simulink model "Thirtybussys"  (R2023b)
settings: Solver=VariableStepAuto  StartTime=0.0  StopTime=1  RelTol=1e-3
libraries: spsFourierLib x60, spsThreePhaseSeriesRLCBranchLib x41, spsThreePhaseVIMeasurementLib x30, spsPower3phInstantaneousLib x30, spsThreePhaseSeriesRLCLoadLib x21, spsThreePhaseSourceLib x6, spsThreePhaseTransformerTwoWindingsLib x6, spsThreePhaseFaultLib x1, sps_lib x1
(part 2 of 2)

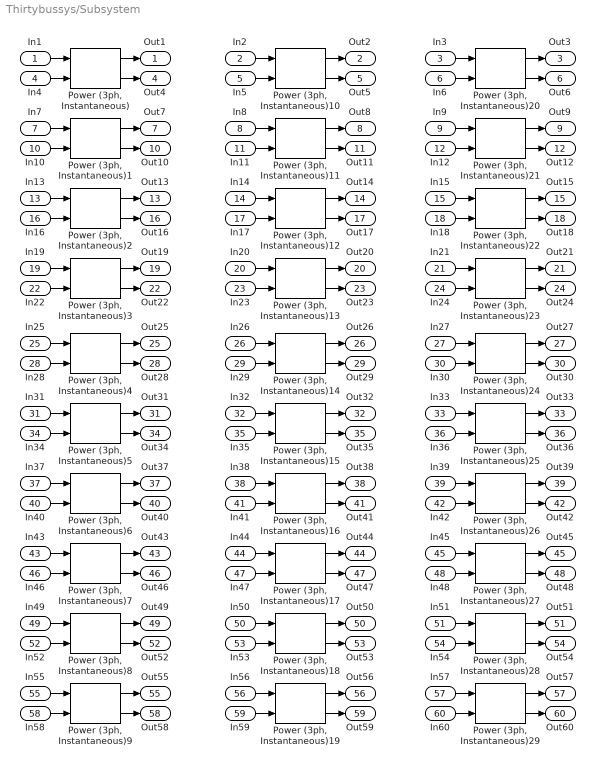
== system Thirtybussys/Subsystem ==
  In1 : Inport
  In2 : Inport  Port=2
  In3 : Inport  Port=3
  In4 : Inport  Port=4
  In5 : Inport  Port=5
  In6 : Inport  Port=6
  In7 : Inport  Port=7
  In8 : Inport  Port=8
  In9 : Inport  Port=9
  In10 : Inport  Port=10
  In11 : Inport  Port=11
  In12 : Inport  Port=12
  In13 : Inport  Port=13
  In14 : Inport  Port=14
  In15 : Inport  Port=15
  In16 : Inport  Port=16
  In17 : Inport  Port=17
  In18 : Inport  Port=18
  In19 : Inport  Port=19
  In20 : Inport  Port=20
  In21 : Inport  Port=21
  In22 : Inport  Port=22
  In23 : Inport  Port=23
  In24 : Inport  Port=24
  In25 : Inport  Port=25
  In26 : Inport  Port=26
  In27 : Inport  Port=27
  In28 : Inport  Port=28
  In29 : Inport  Port=29
  In30 : Inport  Port=30
  In31 : Inport  Port=31
  In32 : Inport  Port=32
  In33 : Inport  Port=33
  In34 : Inport  Port=34
  In35 : Inport  Port=35
  In36 : Inport  Port=36
  In37 : Inport  Port=37
  In38 : Inport  Port=38
  In39 : Inport  Port=39
  In40 : Inport  Port=40
  In41 : Inport  Port=41
  In42 : Inport  Port=42
  In43 : Inport  Port=43
  In44 : Inport  Port=44
  In45 : Inport  Port=45
  In46 : Inport  Port=46
  In47 : Inport  Port=47
  In48 : Inport  Port=48
  In49 : Inport  Port=49
  In50 : Inport  Port=50
  In51 : Inport  Port=51
  In52 : Inport  Port=52
  In53 : Inport  Port=53
  In54 : Inport  Port=54
  In55 : Inport  Port=55
  In56 : Inport  Port=56
  In57 : Inport  Port=57
  In58 : Inport  Port=58
  In59 : Inport  Port=59
  In60 : Inport  Port=60
  Power (3ph, Instantaneous){,1..29} (30 alike) : spsPower3phInstantaneousLib/Power (3ph, Instantaneous)
  Out1 : Outport  VectorParamsAs1DForOutWhenUnconnected=off
  Out2 : Outport  Port=2  VectorParamsAs1DForOutWhenUnconnected=off
  Out3 : Outport  Port=3  VectorParamsAs1DForOutWhenUnconnected=off
  Out4 : Outport  Port=4  VectorParamsAs1DForOutWhenUnconnected=off
  Out5 : Outport  Port=5  VectorParamsAs1DForOutWhenUnconnected=off
  Out6 : Outport  Port=6  VectorParamsAs1DForOutWhenUnconnected=off
  Out7 : Outport  Port=7  VectorParamsAs1DForOutWhenUnconnected=off
  Out8 : Outport  Port=8  VectorParamsAs1DForOutWhenUnconnected=off
  Out9 : Outport  Port=9  VectorParamsAs1DForOutWhenUnconnected=off
  Out10 : Outport  Port=10  VectorParamsAs1DForOutWhenUnconnected=off
  Out11 : Outport  Port=11  VectorParamsAs1DForOutWhenUnconnected=off
  Out12 : Outport  Port=12  VectorParamsAs1DForOutWhenUnconnected=off
  Out13 : Outport  Port=13  VectorParamsAs1DForOutWhenUnconnected=off
  Out14 : Outport  Port=14  VectorParamsAs1DForOutWhenUnconnected=off
  Out15 : Outport  Port=15  VectorParamsAs1DForOutWhenUnconnected=off
  Out16 : Outport  Port=16  VectorParamsAs1DForOutWhenUnconnected=off
  Out17 : Outport  Port=17  VectorParamsAs1DForOutWhenUnconnected=off
  Out18 : Outport  Port=18  VectorParamsAs1DForOutWhenUnconnected=off
  Out19 : Outport  Port=19  VectorParamsAs1DForOutWhenUnconnected=off
  Out20 : Outport  Port=20  VectorParamsAs1DForOutWhenUnconnected=off
  Out21 : Outport  Port=21  VectorParamsAs1DForOutWhenUnconnected=off
  Out22 : Outport  Port=22  VectorParamsAs1DForOutWhenUnconnected=off
  Out23 : Outport  Port=23  VectorParamsAs1DForOutWhenUnconnected=off
  Out24 : Outport  Port=24  VectorParamsAs1DForOutWhenUnconnected=off
  Out25 : Outport  Port=25  VectorParamsAs1DForOutWhenUnconnected=off
  Out26 : Outport  Port=26  VectorParamsAs1DForOutWhenUnconnected=off
  Out27 : Outport  Port=27  VectorParamsAs1DForOutWhenUnconnected=off
  Out28 : Outport  Port=28  VectorParamsAs1DForOutWhenUnconnected=off
  Out29 : Outport  Port=29  VectorParamsAs1DForOutWhenUnconnected=off
  Out30 : Outport  Port=30  VectorParamsAs1DForOutWhenUnconnected=off
  Out31 : Outport  Port=31  VectorParamsAs1DForOutWhenUnconnected=off
  Out32 : Outport  Port=32  VectorParamsAs1DForOutWhenUnconnected=off
  Out33 : Outport  Port=33  VectorParamsAs1DForOutWhenUnconnected=off
  Out34 : Outport  Port=34  VectorParamsAs1DForOutWhenUnconnected=off
  Out35 : Outport  Port=35  VectorParamsAs1DForOutWhenUnconnected=off
  Out36 : Outport  Port=36  VectorParamsAs1DForOutWhenUnconnected=off
  Out37 : Outport  Port=37  VectorParamsAs1DForOutWhenUnconnected=off
  Out38 : Outport  Port=38  VectorParamsAs1DForOutWhenUnconnected=off
  Out39 : Outport  Port=39  VectorParamsAs1DForOutWhenUnconnected=off
  Out40 : Outport  Port=40  VectorParamsAs1DForOutWhenUnconnected=off
  Out41 : Outport  Port=41  VectorParamsAs1DForOutWhenUnconnected=off
  Out42 : Outport  Port=42  VectorParamsAs1DForOutWhenUnconnected=off
  Out43 : Outport  Port=43  VectorParamsAs1DForOutWhenUnconnected=off
  Out44 : Outport  Port=44  VectorParamsAs1DForOutWhenUnconnected=off
  Out45 : Outport  Port=45  VectorParamsAs1DForOutWhenUnconnected=off
  Out46 : Outport  Port=46  VectorParamsAs1DForOutWhenUnconnected=off
  Out47 : Outport  Port=47  VectorParamsAs1DForOutWhenUnconnected=off
  Out48 : Outport  Port=48  VectorParamsAs1DForOutWhenUnconnected=off
  Out49 : Outport  Port=49  VectorParamsAs1DForOutWhenUnconnected=off
  Out50 : Outport  Port=50  VectorParamsAs1DForOutWhenUnconnected=off
  Out51 : Outport  Port=51  VectorParamsAs1DForOutWhenUnconnected=off
  Out52 : Outport  Port=52  VectorParamsAs1DForOutWhenUnconnected=off
  Out53 : Outport  Port=53  VectorParamsAs1DForOutWhenUnconnected=off
  Out54 : Outport  Port=54  VectorParamsAs1DForOutWhenUnconnected=off
  Out55 : Outport  Port=55  VectorParamsAs1DForOutWhenUnconnected=off
  Out56 : Outport  Port=56  VectorParamsAs1DForOutWhenUnconnected=off
  Out57 : Outport  Port=57  VectorParamsAs1DForOutWhenUnconnected=off
  Out58 : Outport  Port=58  VectorParamsAs1DForOutWhenUnconnected=off
  Out59 : Outport  Port=59  VectorParamsAs1DForOutWhenUnconnected=off
  Out60 : Outport  Port=60  VectorParamsAs1DForOutWhenUnconnected=off
  wires:
  In20/1 -> "Power (3ph, Instantaneous)13"/1
  "Power (3ph, Instantaneous)4"/1 -> Out25/1
  In18/1 -> "Power (3ph, Instantaneous)22"/2
  "Power (3ph, Instantaneous)10"/1 -> Out2/1
  "Power (3ph, Instantaneous)11"/2 -> Out11/1
  In48/1 -> "Power (3ph, Instantaneous)27"/2
  "Power (3ph, Instantaneous)28"/2 -> Out54/1
  In25/1 -> "Power (3ph, Instantaneous)4"/1
  In41/1 -> "Power (3ph, Instantaneous)16"/2
  "Power (3ph, Instantaneous)28"/1 -> Out51/1
  In11/1 -> "Power (3ph, Instantaneous)11"/2
  In36/1 -> "Power (3ph, Instantaneous)25"/2
  "Power (3ph, Instantaneous)21"/1 -> Out9/1
  In46/1 -> "Power (3ph, Instantaneous)7"/2
  In38/1 -> "Power (3ph, Instantaneous)16"/1
  "Power (3ph, Instantaneous)14"/2 -> Out29/1
  "Power (3ph, Instantaneous)20"/2 -> Out6/1
  In23/1 -> "Power (3ph, Instantaneous)13"/2
  "Power (3ph, Instantaneous)13"/2 -> Out23/1
  In17/1 -> "Power (3ph, Instantaneous)12"/2
  "Power (3ph, Instantaneous)17"/2 -> Out47/1
  In47/1 -> "Power (3ph, Instantaneous)17"/2
  In26/1 -> "Power (3ph, Instantaneous)14"/1
  "Power (3ph, Instantaneous)15"/1 -> Out32/1
  In12/1 -> "Power (3ph, Instantaneous)21"/2
  "Power (3ph, Instantaneous)8"/2 -> Out52/1
  "Power (3ph, Instantaneous)16"/2 -> Out41/1
  In57/1 -> "Power (3ph, Instantaneous)29"/1
  In35/1 -> "Power (3ph, Instantaneous)15"/2
  In52/1 -> "Power (3ph, Instantaneous)8"/2
  "Power (3ph, Instantaneous)2"/1 -> Out13/1
  In16/1 -> "Power (3ph, Instantaneous)2"/2
  In6/1 -> "Power (3ph, Instantaneous)20"/2
  In29/1 -> "Power (3ph, Instantaneous)14"/2
  In42/1 -> "Power (3ph, Instantaneous)26"/2
  "Power (3ph, Instantaneous)1"/1 -> Out7/1
  In58/1 -> "Power (3ph, Instantaneous)9"/2
  "Power (3ph, Instantaneous)15"/2 -> Out35/1
  In19/1 -> "Power (3ph, Instantaneous)3"/1
  "Power (3ph, Instantaneous)9"/2 -> Out58/1
  In30/1 -> "Power (3ph, Instantaneous)24"/2
  "Power (3ph, Instantaneous)12"/2 -> Out17/1
  "Power (3ph, Instantaneous)24"/2 -> Out30/1
  "Power (3ph, Instantaneous)23"/2 -> Out24/1
  In60/1 -> "Power (3ph, Instantaneous)29"/2
  "Power (3ph, Instantaneous)20"/1 -> Out3/1
  "Power (3ph, Instantaneous)22"/1 -> Out15/1
  In24/1 -> "Power (3ph, Instantaneous)23"/2
  "Power (3ph, Instantaneous)25"/2 -> Out36/1
  In27/1 -> "Power (3ph, Instantaneous)24"/1
  In54/1 -> "Power (3ph, Instantaneous)28"/2
  "Power (3ph, Instantaneous)12"/1 -> Out14/1
  In55/1 -> "Power (3ph, Instantaneous)9"/1
  In22/1 -> "Power (3ph, Instantaneous)3"/2
  "Power (3ph, Instantaneous)2"/2 -> Out16/1
  "Power (3ph, Instantaneous)14"/1 -> Out26/1
  "Power (3ph, Instantaneous)3"/2 -> Out22/1
  "Power (3ph, Instantaneous)26"/2 -> Out42/1
  "Power (3ph, Instantaneous)27"/2 -> Out48/1
  In28/1 -> "Power (3ph, Instantaneous)4"/2
  "Power (3ph, Instantaneous)29"/2 -> Out60/1
  "Power (3ph, Instantaneous)26"/1 -> Out39/1
  "Power (3ph, Instantaneous)23"/1 -> Out21/1
  In7/1 -> "Power (3ph, Instantaneous)1"/1
  "Power (3ph, Instantaneous)7"/2 -> Out46/1
  "Power (3ph, Instantaneous)21"/2 -> Out12/1
  "Power (3ph, Instantaneous)22"/2 -> Out18/1
  In9/1 -> "Power (3ph, Instantaneous)21"/1
  In32/1 -> "Power (3ph, Instantaneous)15"/1
  "Power (3ph, Instantaneous)16"/1 -> Out38/1
  In39/1 -> "Power (3ph, Instantaneous)26"/1
  In15/1 -> "Power (3ph, Instantaneous)22"/1
  In44/1 -> "Power (3ph, Instantaneous)17"/1
  "Power (3ph, Instantaneous)29"/1 -> Out57/1
  "Power (3ph, Instantaneous)24"/1 -> Out27/1
  In21/1 -> "Power (3ph, Instantaneous)23"/1
  In31/1 -> "Power (3ph, Instantaneous)5"/1
  "Power (3ph, Instantaneous)5"/1 -> Out31/1
  In43/1 -> "Power (3ph, Instantaneous)7"/1
  "Power (3ph, Instantaneous)3"/1 -> Out19/1
  "Power (3ph, Instantaneous)6"/1 -> Out37/1
  In37/1 -> "Power (3ph, Instantaneous)6"/1
  In33/1 -> "Power (3ph, Instantaneous)25"/1
  In1/1 -> "Power (3ph, Instantaneous)"/1
  "Power (3ph, Instantaneous)"/1 -> Out1/1
  In50/1 -> "Power (3ph, Instantaneous)18"/1
  "Power (3ph, Instantaneous)25"/1 -> Out33/1
  "Power (3ph, Instantaneous)17"/1 -> Out44/1
  In56/1 -> "Power (3ph, Instantaneous)19"/1
  "Power (3ph, Instantaneous)18"/1 -> Out50/1
  "Power (3ph, Instantaneous)9"/1 -> Out55/1
  "Power (3ph, Instantaneous)7"/1 -> Out43/1
  "Power (3ph, Instantaneous)19"/1 -> Out56/1
  In45/1 -> "Power (3ph, Instantaneous)27"/1
  In2/1 -> "Power (3ph, Instantaneous)10"/1
  In10/1 -> "Power (3ph, Instantaneous)1"/2
  In49/1 -> "Power (3ph, Instantaneous)8"/1
  "Power (3ph, Instantaneous)27"/1 -> Out45/1
  "Power (3ph, Instantaneous)8"/1 -> Out49/1
  "Power (3ph, Instantaneous)13"/1 -> Out20/1
  In14/1 -> "Power (3ph, Instantaneous)12"/1
  In13/1 -> "Power (3ph, Instantaneous)2"/1
  In51/1 -> "Power (3ph, Instantaneous)28"/1
  In3/1 -> "Power (3ph, Instantaneous)20"/1
  In8/1 -> "Power (3ph, Instantaneous)11"/1
  "Power (3ph, Instantaneous)11"/1 -> Out8/1
  "Power (3ph, Instantaneous)"/2 -> Out4/1
  "Power (3ph, Instantaneous)10"/2 -> Out5/1
  "Power (3ph, Instantaneous)4"/2 -> Out28/1
  "Power (3ph, Instantaneous)6"/2 -> Out40/1
  "Power (3ph, Instantaneous)5"/2 -> Out34/1
  "Power (3ph, Instantaneous)18"/2 -> Out53/1
  "Power (3ph, Instantaneous)19"/2 -> Out59/1
  In40/1 -> "Power (3ph, Instantaneous)6"/2
  In53/1 -> "Power (3ph, Instantaneous)18"/2
  In34/1 -> "Power (3ph, Instantaneous)5"/2
  In4/1 -> "Power (3ph, Instantaneous)"/2
  In59/1 -> "Power (3ph, Instantaneous)19"/2
  "Power (3ph, Instantaneous)1"/2 -> Out10/1
  In5/1 -> "Power (3ph, Instantaneous)10"/2

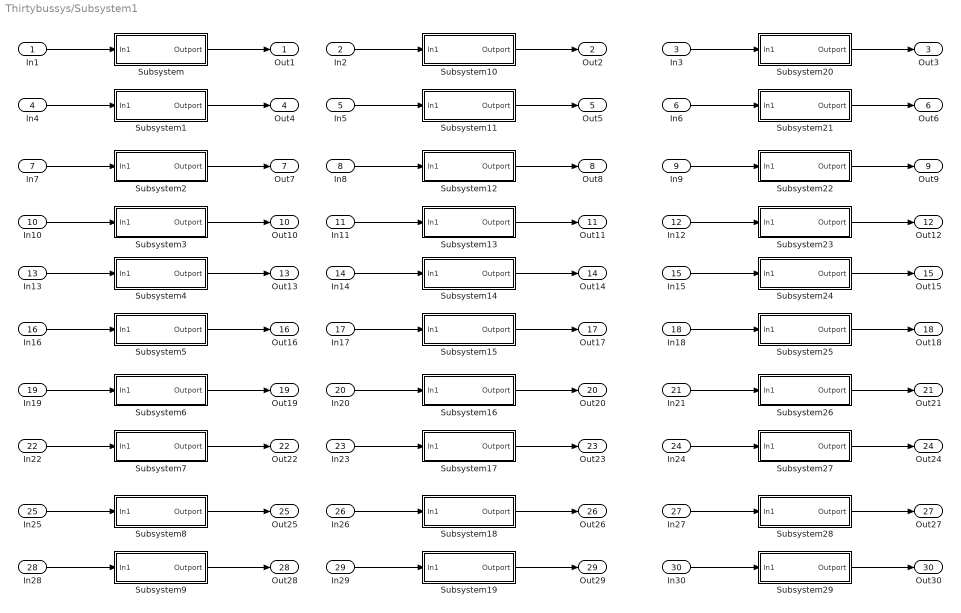
== system Thirtybussys/Subsystem1 ==
  In1 : Inport
  In2 : Inport  Port=2
  In3 : Inport  Port=3
  In4 : Inport  Port=4
  In5 : Inport  Port=5
  In6 : Inport  Port=6
  In7 : Inport  Port=7
  In8 : Inport  Port=8
  In9 : Inport  Port=9
  In10 : Inport  Port=10
  In11 : Inport  Port=11
  In12 : Inport  Port=12
  In13 : Inport  Port=13
  In14 : Inport  Port=14
  In15 : Inport  Port=15
  In16 : Inport  Port=16
  In17 : Inport  Port=17
  In18 : Inport  Port=18
  In19 : Inport  Port=19
  In20 : Inport  Port=20
  In21 : Inport  Port=21
  In22 : Inport  Port=22
  In23 : Inport  Port=23
  In24 : Inport  Port=24
  In25 : Inport  Port=25
  In26 : Inport  Port=26
  In27 : Inport  Port=27
  In28 : Inport  Port=28
  In29 : Inport  Port=29
  In30 : Inport  Port=30
  Subsystem : Subsystem
  Subsystem1 : Subsystem
  Subsystem10 : Subsystem
  Subsystem11 : Subsystem
  Subsystem12 : Subsystem
  Subsystem13 : Subsystem
  Subsystem14 : Subsystem
  Subsystem15 : Subsystem
  Subsystem16 : Subsystem
  Subsystem17 : Subsystem
  Subsystem18 : Subsystem
  Subsystem19 : Subsystem
  Subsystem2 : Subsystem
  Subsystem20 : Subsystem
  Subsystem21 : Subsystem
  Subsystem22 : Subsystem
  Subsystem23 : Subsystem
  Subsystem24 : Subsystem
  Subsystem25 : Subsystem
  Subsystem26 : Subsystem
  Subsystem27 : Subsystem
  Subsystem28 : Subsystem
  Subsystem29 : Subsystem
  Subsystem3 : Subsystem
  Subsystem4 : Subsystem
  Subsystem5 : Subsystem
  Subsystem6 : Subsystem
  Subsystem7 : Subsystem
  Subsystem8 : Subsystem
  Subsystem9 : Subsystem
  Out1 : Outport  VectorParamsAs1DForOutWhenUnconnected=off
  Out2 : Outport  Port=2  VectorParamsAs1DForOutWhenUnconnected=off
  Out3 : Outport  Port=3  VectorParamsAs1DForOutWhenUnconnected=off
  Out4 : Outport  Port=4  VectorParamsAs1DForOutWhenUnconnected=off
  Out5 : Outport  Port=5  VectorParamsAs1DForOutWhenUnconnected=off
  Out6 : Outport  Port=6  VectorParamsAs1DForOutWhenUnconnected=off
  Out7 : Outport  Port=7  VectorParamsAs1DForOutWhenUnconnected=off
  Out8 : Outport  Port=8  VectorParamsAs1DForOutWhenUnconnected=off
  Out9 : Outport  Port=9  VectorParamsAs1DForOutWhenUnconnected=off
  Out10 : Outport  Port=10  VectorParamsAs1DForOutWhenUnconnected=off
  Out11 : Outport  Port=11  VectorParamsAs1DForOutWhenUnconnected=off
  Out12 : Outport  Port=12  VectorParamsAs1DForOutWhenUnconnected=off
  Out13 : Outport  Port=13  VectorParamsAs1DForOutWhenUnconnected=off
  Out14 : Outport  Port=14  VectorParamsAs1DForOutWhenUnconnected=off
  Out15 : Outport  Port=15  VectorParamsAs1DForOutWhenUnconnected=off
  Out16 : Outport  Port=16  VectorParamsAs1DForOutWhenUnconnected=off
  Out17 : Outport  Port=17  VectorParamsAs1DForOutWhenUnconnected=off
  Out18 : Outport  Port=18  VectorParamsAs1DForOutWhenUnconnected=off
  Out19 : Outport  Port=19  VectorParamsAs1DForOutWhenUnconnected=off
  Out20 : Outport  Port=20  VectorParamsAs1DForOutWhenUnconnected=off
  Out21 : Outport  Port=21  VectorParamsAs1DForOutWhenUnconnected=off
  Out22 : Outport  Port=22  VectorParamsAs1DForOutWhenUnconnected=off
  Out23 : Outport  Port=23  VectorParamsAs1DForOutWhenUnconnected=off
  Out24 : Outport  Port=24  VectorParamsAs1DForOutWhenUnconnected=off
  Out25 : Outport  Port=25  VectorParamsAs1DForOutWhenUnconnected=off
  Out26 : Outport  Port=26  VectorParamsAs1DForOutWhenUnconnected=off
  Out27 : Outport  Port=27  VectorParamsAs1DForOutWhenUnconnected=off
  Out28 : Outport  Port=28  VectorParamsAs1DForOutWhenUnconnected=off
  Out29 : Outport  Port=29  VectorParamsAs1DForOutWhenUnconnected=off
  Out30 : Outport  Port=30  VectorParamsAs1DForOutWhenUnconnected=off
  wires:
  Subsystem/1(Outport) -> Out1/1
  Subsystem6/1(Outport) -> Out19/1
  In28/1 -> Subsystem9/1(In1)
  In14/1 -> Subsystem14/1(In1)
  In29/1 -> Subsystem19/1(In1)
  Subsystem7/1(Outport) -> Out22/1
  In11/1 -> Subsystem13/1(In1)
  Subsystem17/1(Outport) -> Out23/1
  In5/1 -> Subsystem11/1(In1)
  Subsystem16/1(Outport) -> Out20/1
  In19/1 -> Subsystem6/1(In1)
  In8/1 -> Subsystem12/1(In1)
  In23/1 -> Subsystem17/1(In1)
  Subsystem18/1(Outport) -> Out26/1
  In25/1 -> Subsystem8/1(In1)
  In10/1 -> Subsystem3/1(In1)
  Subsystem28/1(Outport) -> Out27/1
  In7/1 -> Subsystem2/1(In1)
  Subsystem29/1(Outport) -> Out30/1
  Subsystem15/1(Outport) -> Out17/1
  In26/1 -> Subsystem18/1(In1)
  Subsystem25/1(Outport) -> Out18/1
  In15/1 -> Subsystem24/1(In1)
  Subsystem24/1(Outport) -> Out15/1
  In21/1 -> Subsystem26/1(In1)
  In24/1 -> Subsystem27/1(In1)
  Subsystem1/1(Outport) -> Out4/1
  Subsystem23/1(Outport) -> Out12/1
  Subsystem19/1(Outport) -> Out29/1
  Subsystem13/1(Outport) -> Out11/1
  In3/1 -> Subsystem20/1(In1)
  In12/1 -> Subsystem23/1(In1)
  Subsystem10/1(Outport) -> Out2/1
  In17/1 -> Subsystem15/1(In1)
  In2/1 -> Subsystem10/1(In1)
  Subsystem4/1(Outport) -> Out13/1
  In16/1 -> Subsystem5/1(In1)
  Subsystem14/1(Outport) -> Out14/1
  In13/1 -> Subsystem4/1(In1)
  In18/1 -> Subsystem25/1(In1)
  Subsystem9/1(Outport) -> Out28/1
  Subsystem8/1(Outport) -> Out25/1
  In20/1 -> Subsystem16/1(In1)
  Subsystem20/1(Outport) -> Out3/1
  Subsystem11/1(Outport) -> Out5/1
  Subsystem27/1(Outport) -> Out24/1
  In30/1 -> Subsystem29/1(In1)
  Subsystem2/1(Outport) -> Out7/1
  In22/1 -> Subsystem7/1(In1)
  Subsystem12/1(Outport) -> Out8/1
  Subsystem3/1(Outport) -> Out10/1
  Subsystem21/1(Outport) -> Out6/1
  In9/1 -> Subsystem22/1(In1)
  In4/1 -> Subsystem1/1(In1)
  Subsystem26/1(Outport) -> Out21/1
  Subsystem5/1(Outport) -> Out16/1
  In27/1 -> Subsystem28/1(In1)
  In1/1 -> Subsystem/1(In1)
  In6/1 -> Subsystem21/1(In1)
  Subsystem22/1(Outport) -> Out9/1

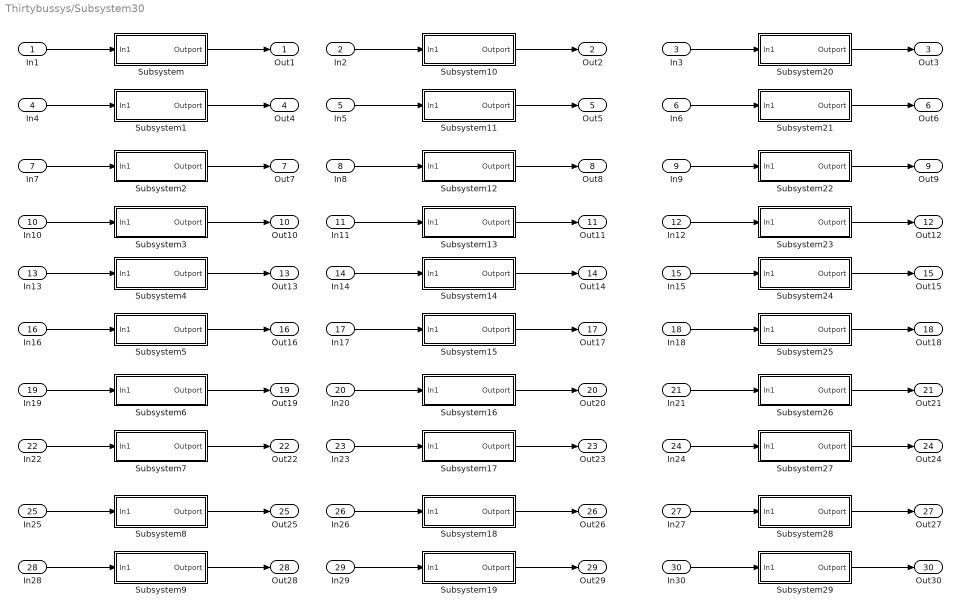
== system Thirtybussys/Subsystem30 ==
  In1 : Inport
  In2 : Inport  Port=2
  In3 : Inport  Port=3
  In4 : Inport  Port=4
  In5 : Inport  Port=5
  In6 : Inport  Port=6
  In7 : Inport  Port=7
  In8 : Inport  Port=8
  In9 : Inport  Port=9
  In10 : Inport  Port=10
  In11 : Inport  Port=11
  In12 : Inport  Port=12
  In13 : Inport  Port=13
  In14 : Inport  Port=14
  In15 : Inport  Port=15
  In16 : Inport  Port=16
  In17 : Inport  Port=17
  In18 : Inport  Port=18
  In19 : Inport  Port=19
  In20 : Inport  Port=20
  In21 : Inport  Port=21
  In22 : Inport  Port=22
  In23 : Inport  Port=23
  In24 : Inport  Port=24
  In25 : Inport  Port=25
  In26 : Inport  Port=26
  In27 : Inport  Port=27
  In28 : Inport  Port=28
  In29 : Inport  Port=29
  In30 : Inport  Port=30
  Subsystem : Subsystem
  Subsystem1 : Subsystem
  Subsystem10 : Subsystem
  Subsystem11 : Subsystem
  Subsystem12 : Subsystem
  Subsystem13 : Subsystem
  Subsystem14 : Subsystem
  Subsystem15 : Subsystem
  Subsystem16 : Subsystem
  Subsystem17 : Subsystem
  Subsystem18 : Subsystem
  Subsystem19 : Subsystem
  Subsystem2 : Subsystem
  Subsystem20 : Subsystem
  Subsystem21 : Subsystem
  Subsystem22 : Subsystem
  Subsystem23 : Subsystem
  Subsystem24 : Subsystem
  Subsystem25 : Subsystem
  Subsystem26 : Subsystem
  Subsystem27 : Subsystem
  Subsystem28 : Subsystem
  Subsystem29 : Subsystem
  Subsystem3 : Subsystem
  Subsystem4 : Subsystem
  Subsystem5 : Subsystem
  Subsystem6 : Subsystem
  Subsystem7 : Subsystem
  Subsystem8 : Subsystem
  Subsystem9 : Subsystem
  Out1 : Outport  VectorParamsAs1DForOutWhenUnconnected=off
  Out2 : Outport  Port=2  VectorParamsAs1DForOutWhenUnconnected=off
  Out3 : Outport  Port=3  VectorParamsAs1DForOutWhenUnconnected=off
  Out4 : Outport  Port=4  VectorParamsAs1DForOutWhenUnconnected=off
  Out5 : Outport  Port=5  VectorParamsAs1DForOutWhenUnconnected=off
  Out6 : Outport  Port=6  VectorParamsAs1DForOutWhenUnconnected=off
  Out7 : Outport  Port=7  VectorParamsAs1DForOutWhenUnconnected=off
  Out8 : Outport  Port=8  VectorParamsAs1DForOutWhenUnconnected=off
  Out9 : Outport  Port=9  VectorParamsAs1DForOutWhenUnconnected=off
  Out10 : Outport  Port=10  VectorParamsAs1DForOutWhenUnconnected=off
  Out11 : Outport  Port=11  VectorParamsAs1DForOutWhenUnconnected=off
  Out12 : Outport  Port=12  VectorParamsAs1DForOutWhenUnconnected=off
  Out13 : Outport  Port=13  VectorParamsAs1DForOutWhenUnconnected=off
  Out14 : Outport  Port=14  VectorParamsAs1DForOutWhenUnconnected=off
  Out15 : Outport  Port=15  VectorParamsAs1DForOutWhenUnconnected=off
  Out16 : Outport  Port=16  VectorParamsAs1DForOutWhenUnconnected=off
  Out17 : Outport  Port=17  VectorParamsAs1DForOutWhenUnconnected=off
  Out18 : Outport  Port=18  VectorParamsAs1DForOutWhenUnconnected=off
  Out19 : Outport  Port=19  VectorParamsAs1DForOutWhenUnconnected=off
  Out20 : Outport  Port=20  VectorParamsAs1DForOutWhenUnconnected=off
  Out21 : Outport  Port=21  VectorParamsAs1DForOutWhenUnconnected=off
  Out22 : Outport  Port=22  VectorParamsAs1DForOutWhenUnconnected=off
  Out23 : Outport  Port=23  VectorParamsAs1DForOutWhenUnconnected=off
  Out24 : Outport  Port=24  VectorParamsAs1DForOutWhenUnconnected=off
  Out25 : Outport  Port=25  VectorParamsAs1DForOutWhenUnconnected=off
  Out26 : Outport  Port=26  VectorParamsAs1DForOutWhenUnconnected=off
  Out27 : Outport  Port=27  VectorParamsAs1DForOutWhenUnconnected=off
  Out28 : Outport  Port=28  VectorParamsAs1DForOutWhenUnconnected=off
  Out29 : Outport  Port=29  VectorParamsAs1DForOutWhenUnconnected=off
  Out30 : Outport  Port=30  VectorParamsAs1DForOutWhenUnconnected=off
  wires:
  Subsystem22/1(Outport) -> Out9/1
  In6/1 -> Subsystem21/1(In1)
  In1/1 -> Subsystem/1(In1)
  In27/1 -> Subsystem28/1(In1)
  Subsystem5/1(Outport) -> Out16/1
  Subsystem26/1(Outport) -> Out21/1
  In4/1 -> Subsystem1/1(In1)
  In9/1 -> Subsystem22/1(In1)
  Subsystem21/1(Outport) -> Out6/1
  Subsystem3/1(Outport) -> Out10/1
  Subsystem12/1(Outport) -> Out8/1
  In22/1 -> Subsystem7/1(In1)
  Subsystem2/1(Outport) -> Out7/1
  In30/1 -> Subsystem29/1(In1)
  Subsystem27/1(Outport) -> Out24/1
  Subsystem11/1(Outport) -> Out5/1
  Subsystem20/1(Outport) -> Out3/1
  In20/1 -> Subsystem16/1(In1)
  Subsystem8/1(Outport) -> Out25/1
  Subsystem9/1(Outport) -> Out28/1
  In18/1 -> Subsystem25/1(In1)
  In13/1 -> Subsystem4/1(In1)
  Subsystem14/1(Outport) -> Out14/1
  In16/1 -> Subsystem5/1(In1)
  Subsystem4/1(Outport) -> Out13/1
  In2/1 -> Subsystem10/1(In1)
  In17/1 -> Subsystem15/1(In1)
  Subsystem10/1(Outport) -> Out2/1
  In12/1 -> Subsystem23/1(In1)
  In3/1 -> Subsystem20/1(In1)
  Subsystem13/1(Outport) -> Out11/1
  Subsystem19/1(Outport) -> Out29/1
  Subsystem23/1(Outport) -> Out12/1
  Subsystem1/1(Outport) -> Out4/1
  In24/1 -> Subsystem27/1(In1)
  In21/1 -> Subsystem26/1(In1)
  Subsystem24/1(Outport) -> Out15/1
  In15/1 -> Subsystem24/1(In1)
  Subsystem25/1(Outport) -> Out18/1
  In26/1 -> Subsystem18/1(In1)
  Subsystem15/1(Outport) -> Out17/1
  Subsystem29/1(Outport) -> Out30/1
  In7/1 -> Subsystem2/1(In1)
  Subsystem28/1(Outport) -> Out27/1
  In10/1 -> Subsystem3/1(In1)
  In25/1 -> Subsystem8/1(In1)
  Subsystem18/1(Outport) -> Out26/1
  In23/1 -> Subsystem17/1(In1)
  In8/1 -> Subsystem12/1(In1)
  In19/1 -> Subsystem6/1(In1)
  Subsystem16/1(Outport) -> Out20/1
  In5/1 -> Subsystem11/1(In1)
  Subsystem17/1(Outport) -> Out23/1
  In11/1 -> Subsystem13/1(In1)
  Subsystem7/1(Outport) -> Out22/1
  In29/1 -> Subsystem19/1(In1)
  In14/1 -> Subsystem14/1(In1)
  In28/1 -> Subsystem9/1(In1)
  Subsystem6/1(Outport) -> Out19/1
  Subsystem/1(Outport) -> Out1/1

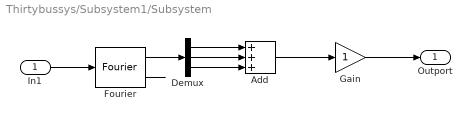
== system Thirtybussys/Subsystem1/Subsystem ==
  In1 : Inport
  Add : Sum  Inputs=+++
  Demux : Demux  Outputs=3
  Fourier : spsFourierLib/Fourier  Freq=60  n=1  InInit=[0, 0]  Ts=0
  Gain : Gain
  Outport : Outport  VectorParamsAs1DForOutWhenUnconnected=off
  wires:
  Demux/1 -> Add/1
  Fourier/1 -> Demux/1
  Demux/2 -> Add/2
  In1/1 -> Fourier/1
  Fourier/2 -> ?
  Gain/1 -> Outport/1
  Add/1 -> Gain/1
  Demux/3 -> Add/3

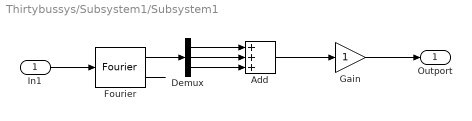
== system Thirtybussys/Subsystem1/Subsystem1 ==
  In1 : Inport
  Add : Sum  Inputs=+++
  Demux : Demux  Outputs=3
  Fourier : spsFourierLib/Fourier  Freq=60  n=1  InInit=[0, 0]  Ts=0
  Gain : Gain
  Outport : Outport  VectorParamsAs1DForOutWhenUnconnected=off
  wires:
  Demux/3 -> Add/3
  Add/1 -> Gain/1
  Gain/1 -> Outport/1
  Fourier/2 -> ?
  In1/1 -> Fourier/1
  Demux/2 -> Add/2
  Fourier/1 -> Demux/1
  Demux/1 -> Add/1

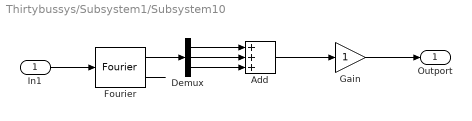
== system Thirtybussys/Subsystem1/Subsystem10 ==
  In1 : Inport
  Add : Sum  Inputs=+++
  Demux : Demux  Outputs=3
  Fourier : spsFourierLib/Fourier  Freq=60  n=1  InInit=[0, 0]  Ts=0
  Gain : Gain
  Outport : Outport  VectorParamsAs1DForOutWhenUnconnected=off
  wires:
  Demux/3 -> Add/3
  Add/1 -> Gain/1
  Gain/1 -> Outport/1
  Fourier/2 -> ?
  In1/1 -> Fourier/1
  Demux/2 -> Add/2
  Fourier/1 -> Demux/1
  Demux/1 -> Add/1

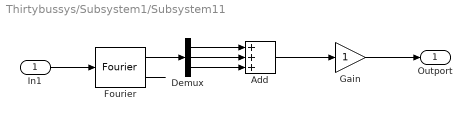
== system Thirtybussys/Subsystem1/Subsystem11 ==
  In1 : Inport
  Add : Sum  Inputs=+++
  Demux : Demux  Outputs=3
  Fourier : spsFourierLib/Fourier  Freq=60  n=1  InInit=[0, 0]  Ts=0
  Gain : Gain
  Outport : Outport  VectorParamsAs1DForOutWhenUnconnected=off
  wires:
  Demux/1 -> Add/1
  Fourier/1 -> Demux/1
  Demux/2 -> Add/2
  In1/1 -> Fourier/1
  Fourier/2 -> ?
  Gain/1 -> Outport/1
  Add/1 -> Gain/1
  Demux/3 -> Add/3

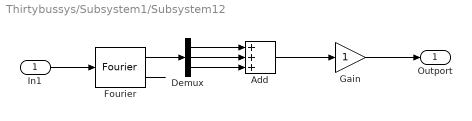
== system Thirtybussys/Subsystem1/Subsystem12 ==
  In1 : Inport
  Add : Sum  Inputs=+++
  Demux : Demux  Outputs=3
  Fourier : spsFourierLib/Fourier  Freq=60  n=1  InInit=[0, 0]  Ts=0
  Gain : Gain
  Outport : Outport  VectorParamsAs1DForOutWhenUnconnected=off
  wires:
  Demux/1 -> Add/1
  Fourier/1 -> Demux/1
  Demux/2 -> Add/2
  In1/1 -> Fourier/1
  Fourier/2 -> ?
  Gain/1 -> Outport/1
  Add/1 -> Gain/1
  Demux/3 -> Add/3

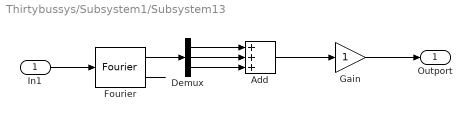
== system Thirtybussys/Subsystem1/Subsystem13 ==
  In1 : Inport
  Add : Sum  Inputs=+++
  Demux : Demux  Outputs=3
  Fourier : spsFourierLib/Fourier  Freq=60  n=1  InInit=[0, 0]  Ts=0
  Gain : Gain
  Outport : Outport  VectorParamsAs1DForOutWhenUnconnected=off
  wires:
  Demux/3 -> Add/3
  Add/1 -> Gain/1
  Gain/1 -> Outport/1
  Fourier/2 -> ?
  In1/1 -> Fourier/1
  Demux/2 -> Add/2
  Fourier/1 -> Demux/1
  Demux/1 -> Add/1

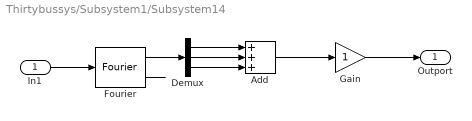
== system Thirtybussys/Subsystem1/Subsystem14 ==
  In1 : Inport
  Add : Sum  Inputs=+++
  Demux : Demux  Outputs=3
  Fourier : spsFourierLib/Fourier  Freq=60  n=1  InInit=[0, 0]  Ts=0
  Gain : Gain
  Outport : Outport  VectorParamsAs1DForOutWhenUnconnected=off
  wires:
  Demux/1 -> Add/1
  Fourier/1 -> Demux/1
  Demux/2 -> Add/2
  In1/1 -> Fourier/1
  Fourier/2 -> ?
  Gain/1 -> Outport/1
  Add/1 -> Gain/1
  Demux/3 -> Add/3

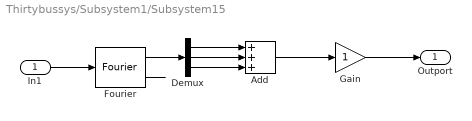
== system Thirtybussys/Subsystem1/Subsystem15 ==
  In1 : Inport
  Add : Sum  Inputs=+++
  Demux : Demux  Outputs=3
  Fourier : spsFourierLib/Fourier  Freq=60  n=1  InInit=[0, 0]  Ts=0
  Gain : Gain
  Outport : Outport  VectorParamsAs1DForOutWhenUnconnected=off
  wires:
  Demux/3 -> Add/3
  Add/1 -> Gain/1
  Gain/1 -> Outport/1
  Fourier/2 -> ?
  In1/1 -> Fourier/1
  Demux/2 -> Add/2
  Fourier/1 -> Demux/1
  Demux/1 -> Add/1

== system Thirtybussys/Subsystem1/Subsystem16 ==
  In1 : Inport
  Add : Sum  Inputs=+++
  Demux : Demux  Outputs=3
  Fourier : spsFourierLib/Fourier  Freq=60  n=1  InInit=[0, 0]  Ts=0
  Gain : Gain
  Outport : Outport  VectorParamsAs1DForOutWhenUnconnected=off
  wires:
  Demux/3 -> Add/3
  Add/1 -> Gain/1
  Gain/1 -> Outport/1
  Fourier/2 -> ?
  In1/1 -> Fourier/1
  Demux/2 -> Add/2
  Fourier/1 -> Demux/1
  Demux/1 -> Add/1

== system Thirtybussys/Subsystem1/Subsystem17 ==
  In1 : Inport
  Add : Sum  Inputs=+++
  Demux : Demux  Outputs=3
  Fourier : spsFourierLib/Fourier  Freq=60  n=1  InInit=[0, 0]  Ts=0
  Gain : Gain
  Outport : Outport  VectorParamsAs1DForOutWhenUnconnected=off
  wires:
  Demux/1 -> Add/1
  Fourier/1 -> Demux/1
  Demux/2 -> Add/2
  In1/1 -> Fourier/1
  Fourier/2 -> ?
  Gain/1 -> Outport/1
  Add/1 -> Gain/1
  Demux/3 -> Add/3

== system Thirtybussys/Subsystem1/Subsystem18 ==
  In1 : Inport
  Add : Sum  Inputs=+++
  Demux : Demux  Outputs=3
  Fourier : spsFourierLib/Fourier  Freq=60  n=1  InInit=[0, 0]  Ts=0
  Gain : Gain
  Outport : Outport  VectorParamsAs1DForOutWhenUnconnected=off
  wires:
  Demux/1 -> Add/1
  Fourier/1 -> Demux/1
  Demux/2 -> Add/2
  In1/1 -> Fourier/1
  Fourier/2 -> ?
  Gain/1 -> Outport/1
  Add/1 -> Gain/1
  Demux/3 -> Add/3

== system Thirtybussys/Subsystem1/Subsystem19 ==
  In1 : Inport
  Add : Sum  Inputs=+++
  Demux : Demux  Outputs=3
  Fourier : spsFourierLib/Fourier  Freq=60  n=1  InInit=[0, 0]  Ts=0
  Gain : Gain
  Outport : Outport  VectorParamsAs1DForOutWhenUnconnected=off
  wires:
  Demux/3 -> Add/3
  Add/1 -> Gain/1
  Gain/1 -> Outport/1
  Fourier/2 -> ?
  In1/1 -> Fourier/1
  Demux/2 -> Add/2
  Fourier/1 -> Demux/1
  Demux/1 -> Add/1

== system Thirtybussys/Subsystem1/Subsystem2 ==
  In1 : Inport
  Add : Sum  Inputs=+++
  Demux : Demux  Outputs=3
  Fourier : spsFourierLib/Fourier  Freq=60  n=1  InInit=[0, 0]  Ts=0
  Gain : Gain
  Outport : Outport  VectorParamsAs1DForOutWhenUnconnected=off
  wires:
  Demux/3 -> Add/3
  Add/1 -> Gain/1
  Gain/1 -> Outport/1
  Fourier/2 -> ?
  In1/1 -> Fourier/1
  Demux/2 -> Add/2
  Fourier/1 -> Demux/1
  Demux/1 -> Add/1

== system Thirtybussys/Subsystem1/Subsystem20 ==
  In1 : Inport
  Add : Sum  Inputs=+++
  Demux : Demux  Outputs=3
  Fourier : spsFourierLib/Fourier  Freq=60  n=1  InInit=[0, 0]  Ts=0
  Gain : Gain
  Outport : Outport  VectorParamsAs1DForOutWhenUnconnected=off
  wires:
  Demux/1 -> Add/1
  Fourier/1 -> Demux/1
  Demux/2 -> Add/2
  In1/1 -> Fourier/1
  Fourier/2 -> ?
  Gain/1 -> Outport/1
  Add/1 -> Gain/1
  Demux/3 -> Add/3

== system Thirtybussys/Subsystem1/Subsystem21 ==
  In1 : Inport
  Add : Sum  Inputs=+++
  Demux : Demux  Outputs=3
  Fourier : spsFourierLib/Fourier  Freq=60  n=1  InInit=[0, 0]  Ts=0
  Gain : Gain
  Outport : Outport  VectorParamsAs1DForOutWhenUnconnected=off
  wires:
  Demux/3 -> Add/3
  Add/1 -> Gain/1
  Gain/1 -> Outport/1
  Fourier/2 -> ?
  In1/1 -> Fourier/1
  Demux/2 -> Add/2
  Fourier/1 -> Demux/1
  Demux/1 -> Add/1

== system Thirtybussys/Subsystem1/Subsystem22 ==
  In1 : Inport
  Add : Sum  Inputs=+++
  Demux : Demux  Outputs=3
  Fourier : spsFourierLib/Fourier  Freq=60  n=1  InInit=[0, 0]  Ts=0
  Gain : Gain
  Outport : Outport  VectorParamsAs1DForOutWhenUnconnected=off
  wires:
  Demux/3 -> Add/3
  Add/1 -> Gain/1
  Gain/1 -> Outport/1
  Fourier/2 -> ?
  In1/1 -> Fourier/1
  Demux/2 -> Add/2
  Fourier/1 -> Demux/1
  Demux/1 -> Add/1

== system Thirtybussys/Subsystem1/Subsystem23 ==
  In1 : Inport
  Add : Sum  Inputs=+++
  Demux : Demux  Outputs=3
  Fourier : spsFourierLib/Fourier  Freq=60  n=1  InInit=[0, 0]  Ts=0
  Gain : Gain
  Outport : Outport  VectorParamsAs1DForOutWhenUnconnected=off
  wires:
  Demux/1 -> Add/1
  Fourier/1 -> Demux/1
  Demux/2 -> Add/2
  In1/1 -> Fourier/1
  Fourier/2 -> ?
  Gain/1 -> Outport/1
  Add/1 -> Gain/1
  Demux/3 -> Add/3

== system Thirtybussys/Subsystem1/Subsystem24 ==
  In1 : Inport
  Add : Sum  Inputs=+++
  Demux : Demux  Outputs=3
  Fourier : spsFourierLib/Fourier  Freq=60  n=1  InInit=[0, 0]  Ts=0
  Gain : Gain
  Outport : Outport  VectorParamsAs1DForOutWhenUnconnected=off
  wires:
  Demux/3 -> Add/3
  Add/1 -> Gain/1
  Gain/1 -> Outport/1
  Fourier/2 -> ?
  In1/1 -> Fourier/1
  Demux/2 -> Add/2
  Fourier/1 -> Demux/1
  Demux/1 -> Add/1

== system Thirtybussys/Subsystem1/Subsystem25 ==
  In1 : Inport
  Add : Sum  Inputs=+++
  Demux : Demux  Outputs=3
  Fourier : spsFourierLib/Fourier  Freq=60  n=1  InInit=[0, 0]  Ts=0
  Gain : Gain
  Outport : Outport  VectorParamsAs1DForOutWhenUnconnected=off
  wires:
  Demux/1 -> Add/1
  Fourier/1 -> Demux/1
  Demux/2 -> Add/2
  In1/1 -> Fourier/1
  Fourier/2 -> ?
  Gain/1 -> Outport/1
  Add/1 -> Gain/1
  Demux/3 -> Add/3

== system Thirtybussys/Subsystem1/Subsystem26 ==
  In1 : Inport
  Add : Sum  Inputs=+++
  Demux : Demux  Outputs=3
  Fourier : spsFourierLib/Fourier  Freq=60  n=1  InInit=[0, 0]  Ts=0
  Gain : Gain
  Outport : Outport  VectorParamsAs1DForOutWhenUnconnected=off
  wires:
  Demux/1 -> Add/1
  Fourier/1 -> Demux/1
  Demux/2 -> Add/2
  In1/1 -> Fourier/1
  Fourier/2 -> ?
  Gain/1 -> Outport/1
  Add/1 -> Gain/1
  Demux/3 -> Add/3

== system Thirtybussys/Subsystem1/Subsystem27 ==
  In1 : Inport
  Add : Sum  Inputs=+++
  Demux : Demux  Outputs=3
  Fourier : spsFourierLib/Fourier  Freq=60  n=1  InInit=[0, 0]  Ts=0
  Gain : Gain
  Outport : Outport  VectorParamsAs1DForOutWhenUnconnected=off
  wires:
  Demux/3 -> Add/3
  Add/1 -> Gain/1
  Gain/1 -> Outport/1
  Fourier/2 -> ?
  In1/1 -> Fourier/1
  Demux/2 -> Add/2
  Fourier/1 -> Demux/1
  Demux/1 -> Add/1

== system Thirtybussys/Subsystem1/Subsystem28 ==
  In1 : Inport
  Add : Sum  Inputs=+++
  Demux : Demux  Outputs=3
  Fourier : spsFourierLib/Fourier  Freq=60  n=1  InInit=[0, 0]  Ts=0
  Gain : Gain
  Outport : Outport  VectorParamsAs1DForOutWhenUnconnected=off
  wires:
  Demux/3 -> Add/3
  Add/1 -> Gain/1
  Gain/1 -> Outport/1
  Fourier/2 -> ?
  In1/1 -> Fourier/1
  Demux/2 -> Add/2
  Fourier/1 -> Demux/1
  Demux/1 -> Add/1

== system Thirtybussys/Subsystem1/Subsystem29 ==
  In1 : Inport
  Add : Sum  Inputs=+++
  Demux : Demux  Outputs=3
  Fourier : spsFourierLib/Fourier  Freq=60  n=1  InInit=[0, 0]  Ts=0
  Gain : Gain
  Outport : Outport  VectorParamsAs1DForOutWhenUnconnected=off
  wires:
  Demux/1 -> Add/1
  Fourier/1 -> Demux/1
  Demux/2 -> Add/2
  In1/1 -> Fourier/1
  Fourier/2 -> ?
  Gain/1 -> Outport/1
  Add/1 -> Gain/1
  Demux/3 -> Add/3

== system Thirtybussys/Subsystem1/Subsystem3 ==
  In1 : Inport
  Add : Sum  Inputs=+++
  Demux : Demux  Outputs=3
  Fourier : spsFourierLib/Fourier  Freq=60  n=1  InInit=[0, 0]  Ts=0
  Gain : Gain
  Outport : Outport  VectorParamsAs1DForOutWhenUnconnected=off
  wires:
  Demux/1 -> Add/1
  Fourier/1 -> Demux/1
  Demux/2 -> Add/2
  In1/1 -> Fourier/1
  Fourier/2 -> ?
  Gain/1 -> Outport/1
  Add/1 -> Gain/1
  Demux/3 -> Add/3

== system Thirtybussys/Subsystem1/Subsystem4 ==
  In1 : Inport
  Add : Sum  Inputs=+++
  Demux : Demux  Outputs=3
  Fourier : spsFourierLib/Fourier  Freq=60  n=1  InInit=[0, 0]  Ts=0
  Gain : Gain
  Outport : Outport  VectorParamsAs1DForOutWhenUnconnected=off
  wires:
  Demux/3 -> Add/3
  Add/1 -> Gain/1
  Gain/1 -> Outport/1
  Fourier/2 -> ?
  In1/1 -> Fourier/1
  Demux/2 -> Add/2
  Fourier/1 -> Demux/1
  Demux/1 -> Add/1

== system Thirtybussys/Subsystem1/Subsystem5 ==
  In1 : Inport
  Add : Sum  Inputs=+++
  Demux : Demux  Outputs=3
  Fourier : spsFourierLib/Fourier  Freq=60  n=1  InInit=[0, 0]  Ts=0
  Gain : Gain
  Outport : Outport  VectorParamsAs1DForOutWhenUnconnected=off
  wires:
  Demux/1 -> Add/1
  Fourier/1 -> Demux/1
  Demux/2 -> Add/2
  In1/1 -> Fourier/1
  Fourier/2 -> ?
  Gain/1 -> Outport/1
  Add/1 -> Gain/1
  Demux/3 -> Add/3

== system Thirtybussys/Subsystem1/Subsystem6 ==
  In1 : Inport
  Add : Sum  Inputs=+++
  Demux : Demux  Outputs=3
  Fourier : spsFourierLib/Fourier  Freq=60  n=1  InInit=[0, 0]  Ts=0
  Gain : Gain
  Outport : Outport  VectorParamsAs1DForOutWhenUnconnected=off
  wires:
  Demux/1 -> Add/1
  Fourier/1 -> Demux/1
  Demux/2 -> Add/2
  In1/1 -> Fourier/1
  Fourier/2 -> ?
  Gain/1 -> Outport/1
  Add/1 -> Gain/1
  Demux/3 -> Add/3

== system Thirtybussys/Subsystem1/Subsystem7 ==
  In1 : Inport
  Add : Sum  Inputs=+++
  Demux : Demux  Outputs=3
  Fourier : spsFourierLib/Fourier  Freq=60  n=1  InInit=[0, 0]  Ts=0
  Gain : Gain
  Outport : Outport  VectorParamsAs1DForOutWhenUnconnected=off
  wires:
  Demux/3 -> Add/3
  Add/1 -> Gain/1
  Gain/1 -> Outport/1
  Fourier/2 -> ?
  In1/1 -> Fourier/1
  Demux/2 -> Add/2
  Fourier/1 -> Demux/1
  Demux/1 -> Add/1

== system Thirtybussys/Subsystem1/Subsystem8 ==
  In1 : Inport
  Add : Sum  Inputs=+++
  Demux : Demux  Outputs=3
  Fourier : spsFourierLib/Fourier  Freq=60  n=1  InInit=[0, 0]  Ts=0
  Gain : Gain
  Outport : Outport  VectorParamsAs1DForOutWhenUnconnected=off
  wires:
  Demux/3 -> Add/3
  Add/1 -> Gain/1
  Gain/1 -> Outport/1
  Fourier/2 -> ?
  In1/1 -> Fourier/1
  Demux/2 -> Add/2
  Fourier/1 -> Demux/1
  Demux/1 -> Add/1

== system Thirtybussys/Subsystem1/Subsystem9 ==
  In1 : Inport
  Add : Sum  Inputs=+++
  Demux : Demux  Outputs=3
  Fourier : spsFourierLib/Fourier  Freq=60  n=1  InInit=[0, 0]  Ts=0
  Gain : Gain
  Outport : Outport  VectorParamsAs1DForOutWhenUnconnected=off
  wires:
  Demux/1 -> Add/1
  Fourier/1 -> Demux/1
  Demux/2 -> Add/2
  In1/1 -> Fourier/1
  Fourier/2 -> ?
  Gain/1 -> Outport/1
  Add/1 -> Gain/1
  Demux/3 -> Add/3

== system Thirtybussys/Subsystem30/Subsystem ==
  In1 : Inport
  Add : Sum  Inputs=+++
  Demux : Demux  Outputs=3
  Fourier : spsFourierLib/Fourier  Freq=60  n=1  InInit=[0, 0]  Ts=0
  Gain : Gain
  Outport : Outport  VectorParamsAs1DForOutWhenUnconnected=off
  wires:
  Demux/3 -> Add/3
  Add/1 -> Gain/1
  Gain/1 -> Outport/1
  Fourier/2 -> ?
  In1/1 -> Fourier/1
  Demux/2 -> Add/2
  Fourier/1 -> Demux/1
  Demux/1 -> Add/1

== system Thirtybussys/Subsystem30/Subsystem1 ==
  In1 : Inport
  Add : Sum  Inputs=+++
  Demux : Demux  Outputs=3
  Fourier : spsFourierLib/Fourier  Freq=60  n=1  InInit=[0, 0]  Ts=0
  Gain : Gain
  Outport : Outport  VectorParamsAs1DForOutWhenUnconnected=off
  wires:
  Demux/1 -> Add/1
  Fourier/1 -> Demux/1
  Demux/2 -> Add/2
  In1/1 -> Fourier/1
  Fourier/2 -> ?
  Gain/1 -> Outport/1
  Add/1 -> Gain/1
  Demux/3 -> Add/3

== system Thirtybussys/Subsystem30/Subsystem10 ==
  In1 : Inport
  Add : Sum  Inputs=+++
  Demux : Demux  Outputs=3
  Fourier : spsFourierLib/Fourier  Freq=60  n=1  InInit=[0, 0]  Ts=0
  Gain : Gain
  Outport : Outport  VectorParamsAs1DForOutWhenUnconnected=off
  wires:
  Demux/1 -> Add/1
  Fourier/1 -> Demux/1
  Demux/2 -> Add/2
  In1/1 -> Fourier/1
  Fourier/2 -> ?
  Gain/1 -> Outport/1
  Add/1 -> Gain/1
  Demux/3 -> Add/3

== system Thirtybussys/Subsystem30/Subsystem11 ==
  In1 : Inport
  Add : Sum  Inputs=+++
  Demux : Demux  Outputs=3
  Fourier : spsFourierLib/Fourier  Freq=60  n=1  InInit=[0, 0]  Ts=0
  Gain : Gain
  Outport : Outport  VectorParamsAs1DForOutWhenUnconnected=off
  wires:
  Demux/3 -> Add/3
  Add/1 -> Gain/1
  Gain/1 -> Outport/1
  Fourier/2 -> ?
  In1/1 -> Fourier/1
  Demux/2 -> Add/2
  Fourier/1 -> Demux/1
  Demux/1 -> Add/1

== system Thirtybussys/Subsystem30/Subsystem12 ==
  In1 : Inport
  Add : Sum  Inputs=+++
  Demux : Demux  Outputs=3
  Fourier : spsFourierLib/Fourier  Freq=60  n=1  InInit=[0, 0]  Ts=0
  Gain : Gain
  Outport : Outport  VectorParamsAs1DForOutWhenUnconnected=off
  wires:
  Demux/3 -> Add/3
  Add/1 -> Gain/1
  Gain/1 -> Outport/1
  Fourier/2 -> ?
  In1/1 -> Fourier/1
  Demux/2 -> Add/2
  Fourier/1 -> Demux/1
  Demux/1 -> Add/1

== system Thirtybussys/Subsystem30/Subsystem13 ==
  In1 : Inport
  Add : Sum  Inputs=+++
  Demux : Demux  Outputs=3
  Fourier : spsFourierLib/Fourier  Freq=60  n=1  InInit=[0, 0]  Ts=0
  Gain : Gain
  Outport : Outport  VectorParamsAs1DForOutWhenUnconnected=off
  wires:
  Demux/1 -> Add/1
  Fourier/1 -> Demux/1
  Demux/2 -> Add/2
  In1/1 -> Fourier/1
  Fourier/2 -> ?
  Gain/1 -> Outport/1
  Add/1 -> Gain/1
  Demux/3 -> Add/3

== system Thirtybussys/Subsystem30/Subsystem14 ==
  In1 : Inport
  Add : Sum  Inputs=+++
  Demux : Demux  Outputs=3
  Fourier : spsFourierLib/Fourier  Freq=60  n=1  InInit=[0, 0]  Ts=0
  Gain : Gain
  Outport : Outport  VectorParamsAs1DForOutWhenUnconnected=off
  wires:
  Demux/3 -> Add/3
  Add/1 -> Gain/1
  Gain/1 -> Outport/1
  Fourier/2 -> ?
  In1/1 -> Fourier/1
  Demux/2 -> Add/2
  Fourier/1 -> Demux/1
  Demux/1 -> Add/1

== system Thirtybussys/Subsystem30/Subsystem15 ==
  In1 : Inport
  Add : Sum  Inputs=+++
  Demux : Demux  Outputs=3
  Fourier : spsFourierLib/Fourier  Freq=60  n=1  InInit=[0, 0]  Ts=0
  Gain : Gain
  Outport : Outport  VectorParamsAs1DForOutWhenUnconnected=off
  wires:
  Demux/1 -> Add/1
  Fourier/1 -> Demux/1
  Demux/2 -> Add/2
  In1/1 -> Fourier/1
  Fourier/2 -> ?
  Gain/1 -> Outport/1
  Add/1 -> Gain/1
  Demux/3 -> Add/3

== system Thirtybussys/Subsystem30/Subsystem16 ==
  In1 : Inport
  Add : Sum  Inputs=+++
  Demux : Demux  Outputs=3
  Fourier : spsFourierLib/Fourier  Freq=60  n=1  InInit=[0, 0]  Ts=0
  Gain : Gain
  Outport : Outport  VectorParamsAs1DForOutWhenUnconnected=off
  wires:
  Demux/1 -> Add/1
  Fourier/1 -> Demux/1
  Demux/2 -> Add/2
  In1/1 -> Fourier/1
  Fourier/2 -> ?
  Gain/1 -> Outport/1
  Add/1 -> Gain/1
  Demux/3 -> Add/3

== system Thirtybussys/Subsystem30/Subsystem17 ==
  In1 : Inport
  Add : Sum  Inputs=+++
  Demux : Demux  Outputs=3
  Fourier : spsFourierLib/Fourier  Freq=60  n=1  InInit=[0, 0]  Ts=0
  Gain : Gain
  Outport : Outport  VectorParamsAs1DForOutWhenUnconnected=off
  wires:
  Demux/3 -> Add/3
  Add/1 -> Gain/1
  Gain/1 -> Outport/1
  Fourier/2 -> ?
  In1/1 -> Fourier/1
  Demux/2 -> Add/2
  Fourier/1 -> Demux/1
  Demux/1 -> Add/1

== system Thirtybussys/Subsystem30/Subsystem18 ==
  In1 : Inport
  Add : Sum  Inputs=+++
  Demux : Demux  Outputs=3
  Fourier : spsFourierLib/Fourier  Freq=60  n=1  InInit=[0, 0]  Ts=0
  Gain : Gain
  Outport : Outport  VectorParamsAs1DForOutWhenUnconnected=off
  wires:
  Demux/3 -> Add/3
  Add/1 -> Gain/1
  Gain/1 -> Outport/1
  Fourier/2 -> ?
  In1/1 -> Fourier/1
  Demux/2 -> Add/2
  Fourier/1 -> Demux/1
  Demux/1 -> Add/1

== system Thirtybussys/Subsystem30/Subsystem19 ==
  In1 : Inport
  Add : Sum  Inputs=+++
  Demux : Demux  Outputs=3
  Fourier : spsFourierLib/Fourier  Freq=60  n=1  InInit=[0, 0]  Ts=0
  Gain : Gain
  Outport : Outport  VectorParamsAs1DForOutWhenUnconnected=off
  wires:
  Demux/1 -> Add/1
  Fourier/1 -> Demux/1
  Demux/2 -> Add/2
  In1/1 -> Fourier/1
  Fourier/2 -> ?
  Gain/1 -> Outport/1
  Add/1 -> Gain/1
  Demux/3 -> Add/3

== system Thirtybussys/Subsystem30/Subsystem2 ==
  In1 : Inport
  Add : Sum  Inputs=+++
  Demux : Demux  Outputs=3
  Fourier : spsFourierLib/Fourier  Freq=60  n=1  InInit=[0, 0]  Ts=0
  Gain : Gain
  Outport : Outport  VectorParamsAs1DForOutWhenUnconnected=off
  wires:
  Demux/1 -> Add/1
  Fourier/1 -> Demux/1
  Demux/2 -> Add/2
  In1/1 -> Fourier/1
  Fourier/2 -> ?
  Gain/1 -> Outport/1
  Add/1 -> Gain/1
  Demux/3 -> Add/3

== system Thirtybussys/Subsystem30/Subsystem20 ==
  In1 : Inport
  Add : Sum  Inputs=+++
  Demux : Demux  Outputs=3
  Fourier : spsFourierLib/Fourier  Freq=60  n=1  InInit=[0, 0]  Ts=0
  Gain : Gain
  Outport : Outport  VectorParamsAs1DForOutWhenUnconnected=off
  wires:
  Demux/3 -> Add/3
  Add/1 -> Gain/1
  Gain/1 -> Outport/1
  Fourier/2 -> ?
  In1/1 -> Fourier/1
  Demux/2 -> Add/2
  Fourier/1 -> Demux/1
  Demux/1 -> Add/1

== system Thirtybussys/Subsystem30/Subsystem21 ==
  In1 : Inport
  Add : Sum  Inputs=+++
  Demux : Demux  Outputs=3
  Fourier : spsFourierLib/Fourier  Freq=60  n=1  InInit=[0, 0]  Ts=0
  Gain : Gain
  Outport : Outport  VectorParamsAs1DForOutWhenUnconnected=off
  wires:
  Demux/1 -> Add/1
  Fourier/1 -> Demux/1
  Demux/2 -> Add/2
  In1/1 -> Fourier/1
  Fourier/2 -> ?
  Gain/1 -> Outport/1
  Add/1 -> Gain/1
  Demux/3 -> Add/3

== system Thirtybussys/Subsystem30/Subsystem22 ==
  In1 : Inport
  Add : Sum  Inputs=+++
  Demux : Demux  Outputs=3
  Fourier : spsFourierLib/Fourier  Freq=60  n=1  InInit=[0, 0]  Ts=0
  Gain : Gain
  Outport : Outport  VectorParamsAs1DForOutWhenUnconnected=off
  wires:
  Demux/1 -> Add/1
  Fourier/1 -> Demux/1
  Demux/2 -> Add/2
  In1/1 -> Fourier/1
  Fourier/2 -> ?
  Gain/1 -> Outport/1
  Add/1 -> Gain/1
  Demux/3 -> Add/3

== system Thirtybussys/Subsystem30/Subsystem23 ==
  In1 : Inport
  Add : Sum  Inputs=+++
  Demux : Demux  Outputs=3
  Fourier : spsFourierLib/Fourier  Freq=60  n=1  InInit=[0, 0]  Ts=0
  Gain : Gain
  Outport : Outport  VectorParamsAs1DForOutWhenUnconnected=off
  wires:
  Demux/3 -> Add/3
  Add/1 -> Gain/1
  Gain/1 -> Outport/1
  Fourier/2 -> ?
  In1/1 -> Fourier/1
  Demux/2 -> Add/2
  Fourier/1 -> Demux/1
  Demux/1 -> Add/1

== system Thirtybussys/Subsystem30/Subsystem24 ==
  In1 : Inport
  Add : Sum  Inputs=+++
  Demux : Demux  Outputs=3
  Fourier : spsFourierLib/Fourier  Freq=60  n=1  InInit=[0, 0]  Ts=0
  Gain : Gain
  Outport : Outport  VectorParamsAs1DForOutWhenUnconnected=off
  wires:
  Demux/1 -> Add/1
  Fourier/1 -> Demux/1
  Demux/2 -> Add/2
  In1/1 -> Fourier/1
  Fourier/2 -> ?
  Gain/1 -> Outport/1
  Add/1 -> Gain/1
  Demux/3 -> Add/3

== system Thirtybussys/Subsystem30/Subsystem25 ==
  In1 : Inport
  Add : Sum  Inputs=+++
  Demux : Demux  Outputs=3
  Fourier : spsFourierLib/Fourier  Freq=60  n=1  InInit=[0, 0]  Ts=0
  Gain : Gain
  Outport : Outport  VectorParamsAs1DForOutWhenUnconnected=off
  wires:
  Demux/3 -> Add/3
  Add/1 -> Gain/1
  Gain/1 -> Outport/1
  Fourier/2 -> ?
  In1/1 -> Fourier/1
  Demux/2 -> Add/2
  Fourier/1 -> Demux/1
  Demux/1 -> Add/1

== system Thirtybussys/Subsystem30/Subsystem26 ==
  In1 : Inport
  Add : Sum  Inputs=+++
  Demux : Demux  Outputs=3
  Fourier : spsFourierLib/Fourier  Freq=60  n=1  InInit=[0, 0]  Ts=0
  Gain : Gain
  Outport : Outport  VectorParamsAs1DForOutWhenUnconnected=off
  wires:
  Demux/3 -> Add/3
  Add/1 -> Gain/1
  Gain/1 -> Outport/1
  Fourier/2 -> ?
  In1/1 -> Fourier/1
  Demux/2 -> Add/2
  Fourier/1 -> Demux/1
  Demux/1 -> Add/1

== system Thirtybussys/Subsystem30/Subsystem27 ==
  In1 : Inport
  Add : Sum  Inputs=+++
  Demux : Demux  Outputs=3
  Fourier : spsFourierLib/Fourier  Freq=60  n=1  InInit=[0, 0]  Ts=0
  Gain : Gain
  Outport : Outport  VectorParamsAs1DForOutWhenUnconnected=off
  wires:
  Demux/1 -> Add/1
  Fourier/1 -> Demux/1
  Demux/2 -> Add/2
  In1/1 -> Fourier/1
  Fourier/2 -> ?
  Gain/1 -> Outport/1
  Add/1 -> Gain/1
  Demux/3 -> Add/3

== system Thirtybussys/Subsystem30/Subsystem28 ==
  In1 : Inport
  Add : Sum  Inputs=+++
  Demux : Demux  Outputs=3
  Fourier : spsFourierLib/Fourier  Freq=60  n=1  InInit=[0, 0]  Ts=0
  Gain : Gain
  Outport : Outport  VectorParamsAs1DForOutWhenUnconnected=off
  wires:
  Demux/1 -> Add/1
  Fourier/1 -> Demux/1
  Demux/2 -> Add/2
  In1/1 -> Fourier/1
  Fourier/2 -> ?
  Gain/1 -> Outport/1
  Add/1 -> Gain/1
  Demux/3 -> Add/3

== system Thirtybussys/Subsystem30/Subsystem29 ==
  In1 : Inport
  Add : Sum  Inputs=+++
  Demux : Demux  Outputs=3
  Fourier : spsFourierLib/Fourier  Freq=60  n=1  InInit=[0, 0]  Ts=0
  Gain : Gain
  Outport : Outport  VectorParamsAs1DForOutWhenUnconnected=off
  wires:
  Demux/3 -> Add/3
  Add/1 -> Gain/1
  Gain/1 -> Outport/1
  Fourier/2 -> ?
  In1/1 -> Fourier/1
  Demux/2 -> Add/2
  Fourier/1 -> Demux/1
  Demux/1 -> Add/1

== system Thirtybussys/Subsystem30/Subsystem3 ==
  In1 : Inport
  Add : Sum  Inputs=+++
  Demux : Demux  Outputs=3
  Fourier : spsFourierLib/Fourier  Freq=60  n=1  InInit=[0, 0]  Ts=0
  Gain : Gain
  Outport : Outport  VectorParamsAs1DForOutWhenUnconnected=off
  wires:
  Demux/3 -> Add/3
  Add/1 -> Gain/1
  Gain/1 -> Outport/1
  Fourier/2 -> ?
  In1/1 -> Fourier/1
  Demux/2 -> Add/2
  Fourier/1 -> Demux/1
  Demux/1 -> Add/1

== system Thirtybussys/Subsystem30/Subsystem4 ==
  In1 : Inport
  Add : Sum  Inputs=+++
  Demux : Demux  Outputs=3
  Fourier : spsFourierLib/Fourier  Freq=60  n=1  InInit=[0, 0]  Ts=0
  Gain : Gain
  Outport : Outport  VectorParamsAs1DForOutWhenUnconnected=off
  wires:
  Demux/1 -> Add/1
  Fourier/1 -> Demux/1
  Demux/2 -> Add/2
  In1/1 -> Fourier/1
  Fourier/2 -> ?
  Gain/1 -> Outport/1
  Add/1 -> Gain/1
  Demux/3 -> Add/3

== system Thirtybussys/Subsystem30/Subsystem5 ==
  In1 : Inport
  Add : Sum  Inputs=+++
  Demux : Demux  Outputs=3
  Fourier : spsFourierLib/Fourier  Freq=60  n=1  InInit=[0, 0]  Ts=0
  Gain : Gain
  Outport : Outport  VectorParamsAs1DForOutWhenUnconnected=off
  wires:
  Demux/3 -> Add/3
  Add/1 -> Gain/1
  Gain/1 -> Outport/1
  Fourier/2 -> ?
  In1/1 -> Fourier/1
  Demux/2 -> Add/2
  Fourier/1 -> Demux/1
  Demux/1 -> Add/1

== system Thirtybussys/Subsystem30/Subsystem6 ==
  In1 : Inport
  Add : Sum  Inputs=+++
  Demux : Demux  Outputs=3
  Fourier : spsFourierLib/Fourier  Freq=60  n=1  InInit=[0, 0]  Ts=0
  Gain : Gain
  Outport : Outport  VectorParamsAs1DForOutWhenUnconnected=off
  wires:
  Demux/3 -> Add/3
  Add/1 -> Gain/1
  Gain/1 -> Outport/1
  Fourier/2 -> ?
  In1/1 -> Fourier/1
  Demux/2 -> Add/2
  Fourier/1 -> Demux/1
  Demux/1 -> Add/1

== system Thirtybussys/Subsystem30/Subsystem7 ==
  In1 : Inport
  Add : Sum  Inputs=+++
  Demux : Demux  Outputs=3
  Fourier : spsFourierLib/Fourier  Freq=60  n=1  InInit=[0, 0]  Ts=0
  Gain : Gain
  Outport : Outport  VectorParamsAs1DForOutWhenUnconnected=off
  wires:
  Demux/1 -> Add/1
  Fourier/1 -> Demux/1
  Demux/2 -> Add/2
  In1/1 -> Fourier/1
  Fourier/2 -> ?
  Gain/1 -> Outport/1
  Add/1 -> Gain/1
  Demux/3 -> Add/3

== system Thirtybussys/Subsystem30/Subsystem8 ==
  In1 : Inport
  Add : Sum  Inputs=+++
  Demux : Demux  Outputs=3
  Fourier : spsFourierLib/Fourier  Freq=60  n=1  InInit=[0, 0]  Ts=0
  Gain : Gain
  Outport : Outport  VectorParamsAs1DForOutWhenUnconnected=off
  wires:
  Demux/1 -> Add/1
  Fourier/1 -> Demux/1
  Demux/2 -> Add/2
  In1/1 -> Fourier/1
  Fourier/2 -> ?
  Gain/1 -> Outport/1
  Add/1 -> Gain/1
  Demux/3 -> Add/3

== system Thirtybussys/Subsystem30/Subsystem9 ==
  In1 : Inport
  Add : Sum  Inputs=+++
  Demux : Demux  Outputs=3
  Fourier : spsFourierLib/Fourier  Freq=60  n=1  InInit=[0, 0]  Ts=0
  Gain : Gain
  Outport : Outport  VectorParamsAs1DForOutWhenUnconnected=off
  wires:
  Demux/3 -> Add/3
  Add/1 -> Gain/1
  Gain/1 -> Outport/1
  Fourier/2 -> ?
  In1/1 -> Fourier/1
  Demux/2 -> Add/2
  Fourier/1 -> Demux/1
  Demux/1 -> Add/1
